simulink library "ammclib_bam_S32K14x"  (R2016a)
settings: Solver=VariableStepAuto  SolverMode=SingleTasking  StartTime=0.0  StopTime=10.0  RelTol=1e-3
undefined symbols (not defined in the file or in its folder): f16A1, f16A2, f16ADCMaxError, f16B0, f16B1, f16B2, f16C1, f16CC1, f16CC1sc, f16CC1sc_D, f16CC1sc_Q, f16CC2, f16CC2sc, f16CC2sc_D, f16CC2sc_Q, f16DerivGain, f16EGain, f16FiltCoef, f16HystOff, f16HystOn, f16IGain, f16IntegGain, f16IntegGainFW, f16IntegGainQ, f16Kd, f16Kq, f16Limit, f16LowerLimit, f16LowerLimit_D, f16LowerLimit_Q, f16LowerLimitFW, f16LowerLimitQ, f16ModIndex, f16OutValOff, f16OutValOn, f16PropGain, f16PropGainFW, f16PropGainQ, f16RampDown, f16RampUp, f16UGain, f16UpperLimit, f16UpperLimit_D, f16UpperLimit_Q, f16UpperLimitFW, f16UpperLimitQ, f16WIGain, f32A1, f32A2, f32ADCMaxError, f32B0, f32B1, f32B2, f32C1, f32CC1, f32CC1sc, f32CC1sc_D, f32CC1sc_Q, f32CC2, f32CC2sc ... (+114)
(part 17 of 22)

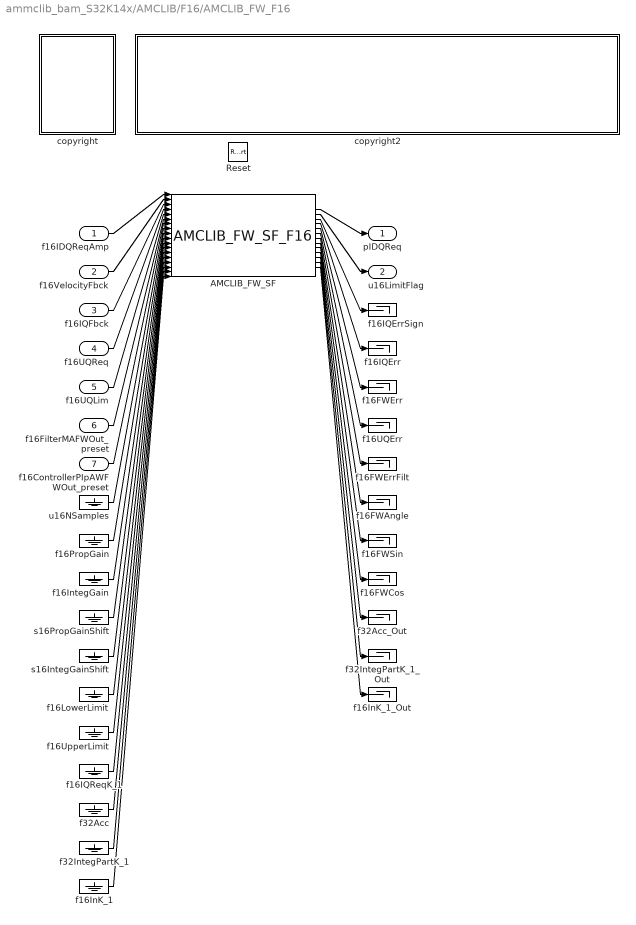
== system ammclib_bam_S32K14x/AMCLIB/F16/AMCLIB_FW_F16 ==
  f16IDQReqAmp : Inport  OutDataTypeStr=int16
  f16VelocityFbck : Inport  Port=2  OutDataTypeStr=int16
  f16IQFbck : Inport  Port=3  OutDataTypeStr=int16
  f16UQReq : Inport  Port=4  OutDataTypeStr=int16
  f16UQLim : Inport  Port=5  OutDataTypeStr=int16
  f16FilterMAFWOut_preset : Inport  Port=6  OutDataTypeStr=int16
  f16ControllerPIpAWFWOut_preset : Inport  Port=7  OutDataTypeStr=int16
  Reset : ResetPort  DisableCoverage=on
  AMCLIB_FW_SF : S-Function  FunctionName=AMCLIB_FW_SF_F16  Parameters=showStates,resetStatesEnable,showDebugOutputs,u16NSamples,f16PropGain,f16IntegGain,s16PropGainShift,s16IntegGainShift,f16LowerLimit,f16UpperLimit  SFunctionDeploymentMode=off  EnableBusSupport=off
  copyright : Subsystem
      mask Display: text(10,90,'FILE:');text(10,75,'DESRIPTION:');text(10,60,'COPYRIGHT:');text(10,45,'VERSION:');text(10,30,'DATE:')
  copyright2 : Subsystem
      mask Display: text(10,90,'AMCLIB_FW_BAM_F16.mdl');text(10,75,'PMSM Field Weakening Controller');text(10,60,'NXP 2020');text(10,45,'1.0');text(10,30,'28-Mar-2020');
  f16FWAngle : Terminator
  f16FWCos : Terminator
  f16FWErr : Terminator
  f16FWErrFilt : Terminator
  f16FWSin : Terminator
  f16IQErr : Terminator
  f16IQErrSign : Terminator
  f16IQReqK_1 : Ground
  f16InK_1 : Ground
  f16InK_1_Out : Terminator
  f16IntegGain : Ground
  f16LowerLimit : Ground
  f16PropGain : Ground
  f16UQErr : Terminator
  f16UpperLimit : Ground
  f32Acc : Ground
  f32Acc_Out : Terminator
  f32IntegPartK_1 : Ground
  f32IntegPartK_1_Out : Terminator
  s16IntegGainShift : Ground
  s16PropGainShift : Ground
  u16NSamples : Ground
  pIDQReq : Outport
  u16LimitFlag : Outport  Port=2
  wires:
  AMCLIB_FW_SF/13 -> f16InK_1_Out/1
  AMCLIB_FW_SF/12 -> f32IntegPartK_1_Out/1
  AMCLIB_FW_SF/11 -> f32Acc_Out/1
  AMCLIB_FW_SF/10 -> f16FWCos/1
  AMCLIB_FW_SF/9 -> f16FWSin/1
  AMCLIB_FW_SF/8 -> f16FWAngle/1
  AMCLIB_FW_SF/7 -> f16FWErrFilt/1
  AMCLIB_FW_SF/6 -> f16UQErr/1
  AMCLIB_FW_SF/5 -> f16FWErr/1
  AMCLIB_FW_SF/4 -> f16IQErr/1
  AMCLIB_FW_SF/3 -> f16IQErrSign/1
  AMCLIB_FW_SF/2 -> u16LimitFlag/1
  AMCLIB_FW_SF/1 -> pIDQReq/1
  f16InK_1/1 -> AMCLIB_FW_SF/18
  f32IntegPartK_1/1 -> AMCLIB_FW_SF/17
  f32Acc/1 -> AMCLIB_FW_SF/16
  f16IQReqK_1/1 -> AMCLIB_FW_SF/15
  f16UpperLimit/1 -> AMCLIB_FW_SF/14
  f16LowerLimit/1 -> AMCLIB_FW_SF/13
  s16IntegGainShift/1 -> AMCLIB_FW_SF/12
  s16PropGainShift/1 -> AMCLIB_FW_SF/11
  f16IntegGain/1 -> AMCLIB_FW_SF/10
  f16PropGain/1 -> AMCLIB_FW_SF/9
  u16NSamples/1 -> AMCLIB_FW_SF/8
  f16ControllerPIpAWFWOut_preset/1 -> AMCLIB_FW_SF/7
  f16FilterMAFWOut_preset/1 -> AMCLIB_FW_SF/6
  f16UQLim/1 -> AMCLIB_FW_SF/5
  f16UQReq/1 -> AMCLIB_FW_SF/4
  f16IQFbck/1 -> AMCLIB_FW_SF/3
  f16VelocityFbck/1 -> AMCLIB_FW_SF/2
  f16IDQReqAmp/1 -> AMCLIB_FW_SF/1

== system ammclib_bam_S32K14x/AMCLIB/F16/AMCLIB_SpeedLoop_F16 ==
  f16VelocityReq : Inport  OutDataTypeStr=int16
  f16VelocityFbck : Inport  Port=2  OutDataTypeStr=int16
  f16FilterMAWOut_preset : Inport  Port=3  OutDataTypeStr=int16
  f16ControllerPIpAWQOut_preset : Inport  Port=4  OutDataTypeStr=int16
  f32RampOut_preset : Inport  Port=5  OutDataTypeStr=int32
  Reset : ResetPort  DisableCoverage=on
  AMCLIB_SpeedLoop_SF : S-Function  FunctionName=AMCLIB_SpeedLoop_SF_F16  Parameters=showStates,resetStatesEnable,showDebugOutputs,u16NSamplesW,f16PropGainQ,f16IntegGainQ,s16PropGainShiftQ,s16IntegGainShiftQ,f16LowerLimitQ,f16UpperLimitQ,f32RampUp,f32RampDown  SFunctionDeploymentMode=off  EnableBusSupport=off
  copyright : Subsystem
      mask Display: text(10,90,'FILE:');text(10,75,'DESRIPTION:');text(10,60,'COPYRIGHT:');text(10,45,'VERSION:');text(10,30,'DATE:')
  copyright2 : Subsystem
      mask Display: text(10,90,'AMCLIB_SpeedLoop_BAM_F16.mdl');text(10,75,'PMSM Speed Loop Controller.');text(10,60,'NXP 2020');text(10,45,'1.0');text(10,30,'28-Mar-2020');
  f16InK_1Q : Ground
  f16InK_1Q_Out : Terminator
  f16IntegGainQ : Ground
  f16LowerLimitQ : Ground
  f16PropGainQ : Ground
  f16UpperLimitQ : Ground
  f16WErr : Terminator
  f16WFbckFilt : Terminator
  f16WReqFilt : Terminator
  f32AccW : Ground
  f32AccW_Out : Terminator
  f32IntegPartK_1Q : Ground
  f32IntegPartK_1Q_Out : Terminator
  f32RampDown : Ground
  f32RampUp : Ground
  f32State : Ground
  f32State_Out : Terminator
  s16IntegGainShiftQ : Ground
  s16PropGainShiftQ : Ground
  u16NSamplesW : Ground
  pIDQReq : Outport
  u16LimitFlagQ : Outport  Port=2
  wires:
  AMCLIB_SpeedLoop_SF/9 -> f32State_Out/1
  AMCLIB_SpeedLoop_SF/8 -> f16InK_1Q_Out/1
  AMCLIB_SpeedLoop_SF/7 -> f32IntegPartK_1Q_Out/1
  AMCLIB_SpeedLoop_SF/6 -> f32AccW_Out/1
  AMCLIB_SpeedLoop_SF/5 -> f16WFbckFilt/1
  AMCLIB_SpeedLoop_SF/4 -> f16WErr/1
  AMCLIB_SpeedLoop_SF/3 -> f16WReqFilt/1
  AMCLIB_SpeedLoop_SF/2 -> u16LimitFlagQ/1
  AMCLIB_SpeedLoop_SF/1 -> pIDQReq/1
  f32State/1 -> AMCLIB_SpeedLoop_SF/18
  f16InK_1Q/1 -> AMCLIB_SpeedLoop_SF/17
  f32IntegPartK_1Q/1 -> AMCLIB_SpeedLoop_SF/16
  f32AccW/1 -> AMCLIB_SpeedLoop_SF/15
  f32RampDown/1 -> AMCLIB_SpeedLoop_SF/14
  f32RampUp/1 -> AMCLIB_SpeedLoop_SF/13
  f16UpperLimitQ/1 -> AMCLIB_SpeedLoop_SF/12
  f16LowerLimitQ/1 -> AMCLIB_SpeedLoop_SF/11
  s16IntegGainShiftQ/1 -> AMCLIB_SpeedLoop_SF/10
  s16PropGainShiftQ/1 -> AMCLIB_SpeedLoop_SF/9
  f16IntegGainQ/1 -> AMCLIB_SpeedLoop_SF/8
  f16PropGainQ/1 -> AMCLIB_SpeedLoop_SF/7
  u16NSamplesW/1 -> AMCLIB_SpeedLoop_SF/6
  f32RampOut_preset/1 -> AMCLIB_SpeedLoop_SF/5
  f16ControllerPIpAWQOut_preset/1 -> AMCLIB_SpeedLoop_SF/4
  f16FilterMAWOut_preset/1 -> AMCLIB_SpeedLoop_SF/3
  f16VelocityFbck/1 -> AMCLIB_SpeedLoop_SF/2
  f16VelocityReq/1 -> AMCLIB_SpeedLoop_SF/1

== system ammclib_bam_S32K14x/AMCLIB/F16/AMCLIB_TrackObsrv_F16 ==
  f16PhaseErr : Inport  OutDataTypeStr=int16
  f16VelocityOut_preset : Inport  Port=2  OutDataTypeStr=int16
  f16PosOut_preset : Inport  Port=3  OutDataTypeStr=int16
  Reset : ResetPort  DisableCoverage=on
  AMCLIB_TrackObsrv_SF : S-Function  FunctionName=AMCLIB_TrackObsrv_SF_F16  Parameters=showStates,resetStatesEnable,f16CC1sc,f16CC2sc,f16UpperLimit,f16LowerLimit,u16NShiftPI,f16C1,u16NShiftI  SFunctionDeploymentMode=off  EnableBusSupport=off
  copyright : Subsystem
      mask Display: text(10,90,'FILE:');text(10,75,'DESRIPTION:');text(10,60,'COPYRIGHT:');text(10,45,'VERSION:');text(10,30,'DATE:')
  copyright2 : Subsystem
      mask Display: text(10,90,'AMCLIB_TrackObsrv_BAM_F16.mdl');text(10,75,'Tracking observer');text(10,60,'NXP 2020');text(10,45,'1.0');text(10,30,'28-Mar-2020');
  f16C1 : Ground
  f16CC1sc : Ground
  f16CC2sc : Ground
  f16InErrK1 : Ground
  f16InErrK1_Out : Terminator
  f16InK1 : Ground
  f16InK1_Out : Terminator
  f16LowerLimit : Ground
  f16UpperLimit : Ground
  f32Acc : Ground
  f32Acc_Out : Terminator
  f32State : Ground
  f32State_Out : Terminator
  u16NShiftI : Ground
  u16NShiftPI : Ground
  pPosEst : Outport
  pVelocityEst : Outport  Port=2
  wires:
  AMCLIB_TrackObsrv_SF/6 -> f16InK1_Out/1
  AMCLIB_TrackObsrv_SF/5 -> f32State_Out/1
  AMCLIB_TrackObsrv_SF/4 -> f16InErrK1_Out/1
  AMCLIB_TrackObsrv_SF/3 -> f32Acc_Out/1
  AMCLIB_TrackObsrv_SF/2 -> pVelocityEst/1
  AMCLIB_TrackObsrv_SF/1 -> pPosEst/1
  f16InK1/1 -> AMCLIB_TrackObsrv_SF/14
  f32State/1 -> AMCLIB_TrackObsrv_SF/13
  f16InErrK1/1 -> AMCLIB_TrackObsrv_SF/12
  f32Acc/1 -> AMCLIB_TrackObsrv_SF/11
  u16NShiftI/1 -> AMCLIB_TrackObsrv_SF/10
  f16C1/1 -> AMCLIB_TrackObsrv_SF/9
  u16NShiftPI/1 -> AMCLIB_TrackObsrv_SF/8
  f16LowerLimit/1 -> AMCLIB_TrackObsrv_SF/7
  f16UpperLimit/1 -> AMCLIB_TrackObsrv_SF/6
  f16CC2sc/1 -> AMCLIB_TrackObsrv_SF/5
  f16CC1sc/1 -> AMCLIB_TrackObsrv_SF/4
  f16PosOut_preset/1 -> AMCLIB_TrackObsrv_SF/3
  f16VelocityOut_preset/1 -> AMCLIB_TrackObsrv_SF/2
  f16PhaseErr/1 -> AMCLIB_TrackObsrv_SF/1

== system ammclib_bam_S32K14x/AMCLIB/F16/AMCLIB_Windmilling_F16 ==
  pUabcIn : Inport  OutDataTypeStr=Bus: SWLIBS_3Syst_F16  BusOutputAsStruct=on
  AMCLIB_Windmilling_SF : S-Function  FunctionName=AMCLIB_Windmilling_SF_F16  Parameters=showStates,f16ADCMaxError,f16CC1sc,f16CC2sc,f16UpperLimit,f16LowerLimit,u16NShiftPI,f16C1,u16NShiftI  SFunctionDeploymentMode=off  EnableBusSupport=off
  copyright : Subsystem
      mask Display: text(10,90,'FILE:');text(10,75,'DESRIPTION:');text(10,60,'COPYRIGHT:');text(10,45,'VERSION:');text(10,30,'DATE:')
  copyright2 : Subsystem
      mask Display: text(10,90,'AMCLIB_Windmilling_BAM_F16.mdl');text(10,75,'PMSM Windmilling');text(10,60,'NXP 2020');text(10,45,'1.0');text(10,30,'28-Mar-2020');
  f16ADCMaxError : Ground
  f16C1 : Ground
  f16CC1sc : Ground
  f16CC2sc : Ground
  f16InErrK1 : Ground
  f16InErrK1_Out : Terminator
  f16InK1 : Ground
  f16InK1_Out : Terminator
  f16LowerLimit : Ground
  f16UpperLimit : Ground
  f32AccPI : Ground
  f32AccPI_Out : Terminator
  f32State : Ground
  f32State_Out : Terminator
  u16NShiftI : Ground
  u16NShiftPI : Ground
  u16Lock : Outport
  pPosEst : Outport  Port=2
  pVelocityEst : Outport  Port=3
  wires:
  AMCLIB_Windmilling_SF/7 -> f16InK1_Out/1
  AMCLIB_Windmilling_SF/6 -> f32State_Out/1
  AMCLIB_Windmilling_SF/5 -> f16InErrK1_Out/1
  AMCLIB_Windmilling_SF/4 -> f32AccPI_Out/1
  AMCLIB_Windmilling_SF/3 -> pVelocityEst/1
  AMCLIB_Windmilling_SF/2 -> pPosEst/1
  AMCLIB_Windmilling_SF/1 -> u16Lock/1
  f16InK1/1 -> AMCLIB_Windmilling_SF/13
  f32State/1 -> AMCLIB_Windmilling_SF/12
  f16InErrK1/1 -> AMCLIB_Windmilling_SF/11
  f32AccPI/1 -> AMCLIB_Windmilling_SF/10
  u16NShiftI/1 -> AMCLIB_Windmilling_SF/9
  f16C1/1 -> AMCLIB_Windmilling_SF/8
  u16NShiftPI/1 -> AMCLIB_Windmilling_SF/7
  f16LowerLimit/1 -> AMCLIB_Windmilling_SF/6
  f16UpperLimit/1 -> AMCLIB_Windmilling_SF/5
  f16CC2sc/1 -> AMCLIB_Windmilling_SF/4
  f16CC1sc/1 -> AMCLIB_Windmilling_SF/3
  f16ADCMaxError/1 -> AMCLIB_Windmilling_SF/2
  pUabcIn/1 -> AMCLIB_Windmilling_SF/1

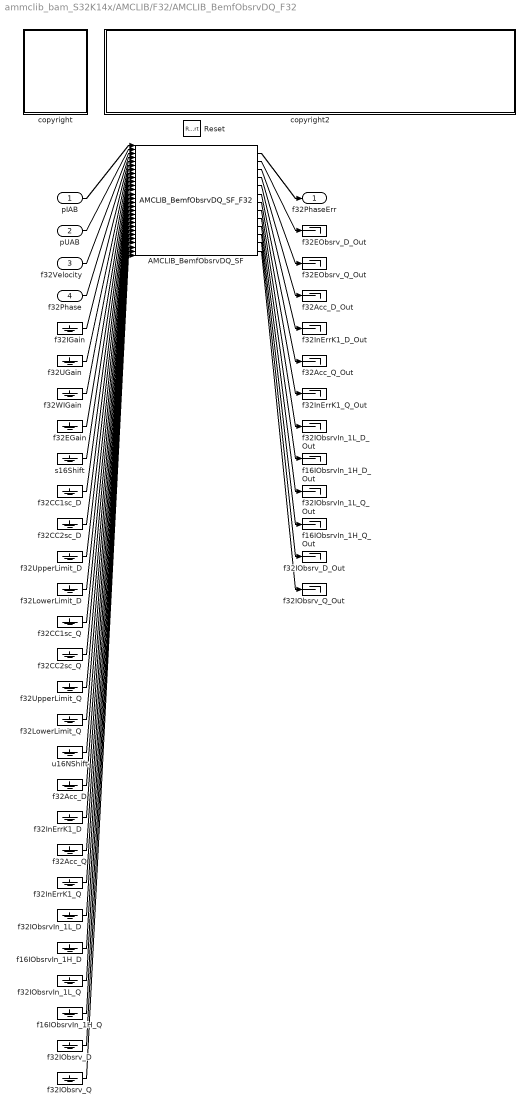
== system ammclib_bam_S32K14x/AMCLIB/F32/AMCLIB_BemfObsrvDQ_F32 ==
  pIAB : Inport  OutDataTypeStr=Bus: SWLIBS_2Syst_F32  BusOutputAsStruct=on
  pUAB : Inport  Port=2  OutDataTypeStr=Bus: SWLIBS_2Syst_F32  BusOutputAsStruct=on
  f32Velocity : Inport  Port=3  OutDataTypeStr=int32
  f32Phase : Inport  Port=4  OutDataTypeStr=int32
  Reset : ResetPort  DisableCoverage=on
  AMCLIB_BemfObsrvDQ_SF : S-Function  FunctionName=AMCLIB_BemfObsrvDQ_SF_F32  Parameters=showStates,resetStatesEnable,f32IGain,f32UGain,f32WIGain,f32EGain,s16Shift,f32CC1sc_D,f32CC2sc_D,f32UpperLimit_D,f32LowerLimit_D,f32CC1sc_Q,f32CC2sc_Q,f32UpperLimit_Q,f32LowerLimit_Q,u16NShift  SFunctionDeploymentMode=off  EnableBusSupport=off
  copyright : Subsystem
      mask Display: text(10,90,'FILE:');text(10,75,'DESRIPTION:');text(10,60,'COPYRIGHT:');text(10,45,'VERSION:');text(10,30,'DATE:')
  copyright2 : Subsystem
      mask Display: text(10,90,'AMCLIB_BemfObsrvDQ_BAM_F32.mdl');text(10,75,'PMSM back-EMF observer DQ.');text(10,60,'NXP 2020');text(10,45,'1.0');text(10,30,'28-Mar-2020');
  f16IObsrvIn_1H_D : Ground
  f16IObsrvIn_1H_D_Out : Terminator
  f16IObsrvIn_1H_Q : Ground
  f16IObsrvIn_1H_Q_Out : Terminator
  f32Acc_D : Ground
  f32Acc_D_Out : Terminator
  f32Acc_Q : Ground
  f32Acc_Q_Out : Terminator
  f32CC1sc_D : Ground
  f32CC1sc_Q : Ground
  f32CC2sc_D : Ground
  f32CC2sc_Q : Ground
  f32EGain : Ground
  f32EObsrv_D_Out : Terminator
  f32EObsrv_Q_Out : Terminator
  f32IGain : Ground
  f32IObsrvIn_1L_D : Ground
  f32IObsrvIn_1L_D_Out : Terminator
  f32IObsrvIn_1L_Q : Ground
  f32IObsrvIn_1L_Q_Out : Terminator
  f32IObsrv_D : Ground
  f32IObsrv_D_Out : Terminator
  f32IObsrv_Q : Ground
  f32IObsrv_Q_Out : Terminator
  f32InErrK1_D : Ground
  f32InErrK1_D_Out : Terminator
  f32InErrK1_Q : Ground
  f32InErrK1_Q_Out : Terminator
  f32LowerLimit_D : Ground
  f32LowerLimit_Q : Ground
  f32UGain : Ground
  f32UpperLimit_D : Ground
  f32UpperLimit_Q : Ground
  f32WIGain : Ground
  s16Shift : Ground
  u16NShift : Ground
  f32PhaseErr : Outport
  wires:
  AMCLIB_BemfObsrvDQ_SF/13 -> f32IObsrv_Q_Out/1
  AMCLIB_BemfObsrvDQ_SF/12 -> f32IObsrv_D_Out/1
  AMCLIB_BemfObsrvDQ_SF/11 -> f16IObsrvIn_1H_Q_Out/1
  AMCLIB_BemfObsrvDQ_SF/10 -> f32IObsrvIn_1L_Q_Out/1
  AMCLIB_BemfObsrvDQ_SF/9 -> f16IObsrvIn_1H_D_Out/1
  AMCLIB_BemfObsrvDQ_SF/8 -> f32IObsrvIn_1L_D_Out/1
  AMCLIB_BemfObsrvDQ_SF/7 -> f32InErrK1_Q_Out/1
  AMCLIB_BemfObsrvDQ_SF/6 -> f32Acc_Q_Out/1
  AMCLIB_BemfObsrvDQ_SF/5 -> f32InErrK1_D_Out/1
  AMCLIB_BemfObsrvDQ_SF/4 -> f32Acc_D_Out/1
  AMCLIB_BemfObsrvDQ_SF/3 -> f32EObsrv_Q_Out/1
  AMCLIB_BemfObsrvDQ_SF/2 -> f32EObsrv_D_Out/1
  AMCLIB_BemfObsrvDQ_SF/1 -> f32PhaseErr/1
  f32IObsrv_Q/1 -> AMCLIB_BemfObsrvDQ_SF/28
  f32IObsrv_D/1 -> AMCLIB_BemfObsrvDQ_SF/27
  f16IObsrvIn_1H_Q/1 -> AMCLIB_BemfObsrvDQ_SF/26
  f32IObsrvIn_1L_Q/1 -> AMCLIB_BemfObsrvDQ_SF/25
  f16IObsrvIn_1H_D/1 -> AMCLIB_BemfObsrvDQ_SF/24
  f32IObsrvIn_1L_D/1 -> AMCLIB_BemfObsrvDQ_SF/23
  f32InErrK1_Q/1 -> AMCLIB_BemfObsrvDQ_SF/22
  f32Acc_Q/1 -> AMCLIB_BemfObsrvDQ_SF/21
  f32InErrK1_D/1 -> AMCLIB_BemfObsrvDQ_SF/20
  f32Acc_D/1 -> AMCLIB_BemfObsrvDQ_SF/19
  u16NShift/1 -> AMCLIB_BemfObsrvDQ_SF/18
  f32LowerLimit_Q/1 -> AMCLIB_BemfObsrvDQ_SF/17
  f32UpperLimit_Q/1 -> AMCLIB_BemfObsrvDQ_SF/16
  f32CC2sc_Q/1 -> AMCLIB_BemfObsrvDQ_SF/15
  f32CC1sc_Q/1 -> AMCLIB_BemfObsrvDQ_SF/14
  f32LowerLimit_D/1 -> AMCLIB_BemfObsrvDQ_SF/13
  f32UpperLimit_D/1 -> AMCLIB_BemfObsrvDQ_SF/12
  f32CC2sc_D/1 -> AMCLIB_BemfObsrvDQ_SF/11
  f32CC1sc_D/1 -> AMCLIB_BemfObsrvDQ_SF/10
  s16Shift/1 -> AMCLIB_BemfObsrvDQ_SF/9
  f32EGain/1 -> AMCLIB_BemfObsrvDQ_SF/8
  f32WIGain/1 -> AMCLIB_BemfObsrvDQ_SF/7
  f32UGain/1 -> AMCLIB_BemfObsrvDQ_SF/6
  f32IGain/1 -> AMCLIB_BemfObsrvDQ_SF/5
  f32Phase/1 -> AMCLIB_BemfObsrvDQ_SF/4
  f32Velocity/1 -> AMCLIB_BemfObsrvDQ_SF/3
  pUAB/1 -> AMCLIB_BemfObsrvDQ_SF/2
  pIAB/1 -> AMCLIB_BemfObsrvDQ_SF/1

== system ammclib_bam_S32K14x/AMCLIB/F32/AMCLIB_CurrentLoop_F32 ==
  f32UDcBus : Inport  OutDataTypeStr=int32
  pIDQReq : Inport  Port=2  OutDataTypeStr=Bus: SWLIBS_2Syst_F32  BusOutputAsStruct=on
  pIDQFbck : Inport  Port=3  OutDataTypeStr=Bus: SWLIBS_2Syst_F32  BusOutputAsStruct=on
  f32ControllerPIrAWDOut_preset : Inport  Port=4  OutDataTypeStr=int32
  f32ControllerPIrAWQOut_preset : Inport  Port=5  OutDataTypeStr=int32
  Reset : ResetPort  DisableCoverage=on
  AMCLIB_CurrentLoop_SF : S-Function  FunctionName=AMCLIB_CurrentLoop_SF_F32  Parameters=showStates,resetStatesEnable,f32CC1sc_D,f32CC2sc_D,u16NShift_D,f32CC1sc_Q,f32CC2sc_Q,u16NShift_Q  SFunctionDeploymentMode=off  EnableBusSupport=off
  copyright : Subsystem
      mask Display: text(10,90,'FILE:');text(10,75,'DESRIPTION:');text(10,60,'COPYRIGHT:');text(10,45,'VERSION:');text(10,30,'DATE:')
  copyright2 : Subsystem
      mask Display: text(10,90,'AMCLIB_CurrentLoop_BAM_F32.mdl');text(10,75,'PMSM Current Loop.');text(10,60,'NXP 2020');text(10,45,'1.0');text(10,30,'28-Mar-2020');
  f32Acc_D : Ground
  f32Acc_D_Out : Terminator
  f32Acc_Q : Ground
  f32Acc_Q_Out : Terminator
  f32CC1sc_D : Ground
  f32CC1sc_Q : Ground
  f32CC2sc_D : Ground
  f32CC2sc_Q : Ground
  f32InErrK1_D : Ground
  f32InErrK1_D_Out : Terminator
  f32InErrK1_Q : Ground
  f32InErrK1_Q_Out : Terminator
  u16NShift_D : Ground
  u16NShift_Q : Ground
  pUDQReq : Outport
  wires:
  AMCLIB_CurrentLoop_SF/5 -> f32InErrK1_Q_Out/1
  AMCLIB_CurrentLoop_SF/4 -> f32Acc_Q_Out/1
  AMCLIB_CurrentLoop_SF/3 -> f32InErrK1_D_Out/1
  AMCLIB_CurrentLoop_SF/2 -> f32Acc_D_Out/1
  AMCLIB_CurrentLoop_SF/1 -> pUDQReq/1
  f32InErrK1_Q/1 -> AMCLIB_CurrentLoop_SF/15
  f32Acc_Q/1 -> AMCLIB_CurrentLoop_SF/14
  f32InErrK1_D/1 -> AMCLIB_CurrentLoop_SF/13
  f32Acc_D/1 -> AMCLIB_CurrentLoop_SF/12
  u16NShift_Q/1 -> AMCLIB_CurrentLoop_SF/11
  f32CC2sc_Q/1 -> AMCLIB_CurrentLoop_SF/10
  f32CC1sc_Q/1 -> AMCLIB_CurrentLoop_SF/9
  u16NShift_D/1 -> AMCLIB_CurrentLoop_SF/8
  f32CC2sc_D/1 -> AMCLIB_CurrentLoop_SF/7
  f32CC1sc_D/1 -> AMCLIB_CurrentLoop_SF/6
  f32ControllerPIrAWQOut_preset/1 -> AMCLIB_CurrentLoop_SF/5
  f32ControllerPIrAWDOut_preset/1 -> AMCLIB_CurrentLoop_SF/4
  pIDQFbck/1 -> AMCLIB_CurrentLoop_SF/3
  pIDQReq/1 -> AMCLIB_CurrentLoop_SF/2
  f32UDcBus/1 -> AMCLIB_CurrentLoop_SF/1

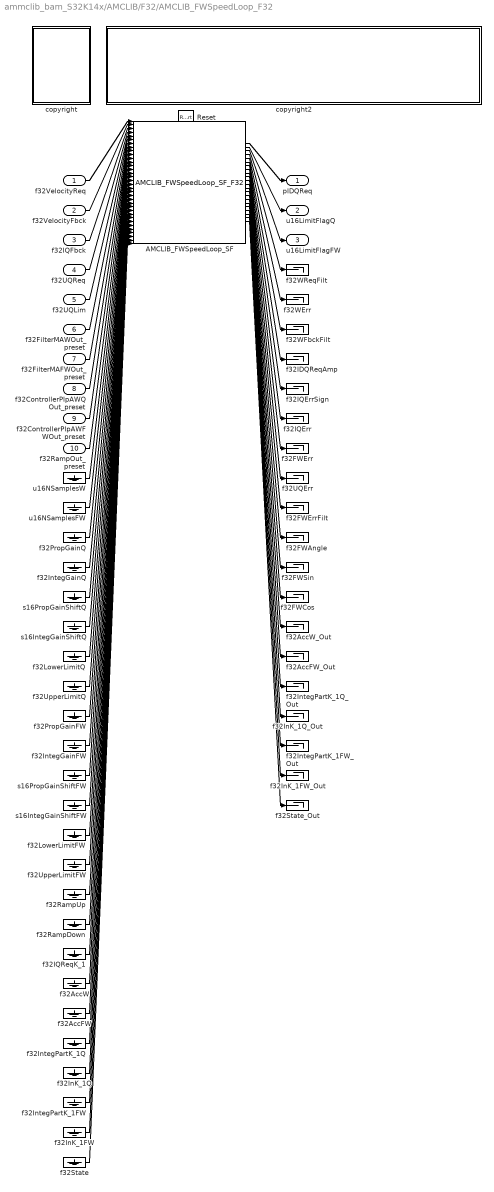
== system ammclib_bam_S32K14x/AMCLIB/F32/AMCLIB_FWSpeedLoop_F32 ==
  f32VelocityReq : Inport  OutDataTypeStr=int32
  f32VelocityFbck : Inport  Port=2  OutDataTypeStr=int32
  f32IQFbck : Inport  Port=3  OutDataTypeStr=int32
  f32UQReq : Inport  Port=4  OutDataTypeStr=int32
  f32UQLim : Inport  Port=5  OutDataTypeStr=int32
  f32FilterMAWOut_preset : Inport  Port=6  OutDataTypeStr=int32
  f32FilterMAFWOut_preset : Inport  Port=7  OutDataTypeStr=int32
  f32ControllerPIpAWQOut_preset : Inport  Port=8  OutDataTypeStr=int32
  f32ControllerPIpAWFWOut_preset : Inport  Port=9  OutDataTypeStr=int32
  f32RampOut_preset : Inport  Port=10  OutDataTypeStr=int32
  Reset : ResetPort  DisableCoverage=on
  AMCLIB_FWSpeedLoop_SF : S-Function  FunctionName=AMCLIB_FWSpeedLoop_SF_F32  Parameters=showStates,resetStatesEnable,showDebugOutputs,u16NSamplesW,u16NSamplesFW,f32PropGainQ,f32IntegGainQ,s16PropGainShiftQ,s16IntegGainShiftQ,f32LowerLimitQ,f32UpperLimitQ,f32PropGainFW,f32IntegGainFW,s16PropGainShiftFW,s16IntegGainShiftFW,f32LowerLimitFW,f32UpperLimitFW,f32RampUp,f32RampDown  SFunctionDeploymentMode=off  EnableBusSupport=off
  copyright : Subsystem
      mask Display: text(10,90,'FILE:');text(10,75,'DESRIPTION:');text(10,60,'COPYRIGHT:');text(10,45,'VERSION:');text(10,30,'DATE:')
  copyright2 : Subsystem
      mask Display: text(10,90,'AMCLIB_FWSpeedLoop_BAM_F32.mdl');text(10,75,'PMSM Speed Loop with Field Weakening.');text(10,60,'NXP 2020');text(10,45,'1.0');text(10,30,'28-Mar-2020');
  f32AccFW : Ground
  f32AccFW_Out : Terminator
  f32AccW : Ground
  f32AccW_Out : Terminator
  f32FWAngle : Terminator
  f32FWCos : Terminator
  f32FWErr : Terminator
  f32FWErrFilt : Terminator
  f32FWSin : Terminator
  f32IDQReqAmp : Terminator
  f32IQErr : Terminator
  f32IQErrSign : Terminator
  f32IQReqK_1 : Ground
  f32InK_1FW : Ground
  f32InK_1FW_Out : Terminator
  f32InK_1Q : Ground
  f32InK_1Q_Out : Terminator
  f32IntegGainFW : Ground
  f32IntegGainQ : Ground
  f32IntegPartK_1FW : Ground
  f32IntegPartK_1FW_Out : Terminator
  f32IntegPartK_1Q : Ground
  f32IntegPartK_1Q_Out : Terminator
  f32LowerLimitFW : Ground
  f32LowerLimitQ : Ground
  f32PropGainFW : Ground
  f32PropGainQ : Ground
  f32RampDown : Ground
  f32RampUp : Ground
  f32State : Ground
  f32State_Out : Terminator
  f32UQErr : Terminator
  f32UpperLimitFW : Ground
  f32UpperLimitQ : Ground
  f32WErr : Terminator
  f32WFbckFilt : Terminator
  f32WReqFilt : Terminator
  s16IntegGainShiftFW : Ground
  s16IntegGainShiftQ : Ground
  s16PropGainShiftFW : Ground
  s16PropGainShiftQ : Ground
  u16NSamplesFW : Ground
  u16NSamplesW : Ground
  pIDQReq : Outport
  u16LimitFlagQ : Outport  Port=2
  u16LimitFlagFW : Outport  Port=3
  wires:
  AMCLIB_FWSpeedLoop_SF/22 -> f32State_Out/1
  AMCLIB_FWSpeedLoop_SF/21 -> f32InK_1FW_Out/1
  AMCLIB_FWSpeedLoop_SF/20 -> f32IntegPartK_1FW_Out/1
  AMCLIB_FWSpeedLoop_SF/19 -> f32InK_1Q_Out/1
  AMCLIB_FWSpeedLoop_SF/18 -> f32IntegPartK_1Q_Out/1
  AMCLIB_FWSpeedLoop_SF/17 -> f32AccFW_Out/1
  AMCLIB_FWSpeedLoop_SF/16 -> f32AccW_Out/1
  AMCLIB_FWSpeedLoop_SF/15 -> f32FWCos/1
  AMCLIB_FWSpeedLoop_SF/14 -> f32FWSin/1
  AMCLIB_FWSpeedLoop_SF/13 -> f32FWAngle/1
  AMCLIB_FWSpeedLoop_SF/12 -> f32FWErrFilt/1
  AMCLIB_FWSpeedLoop_SF/11 -> f32UQErr/1
  AMCLIB_FWSpeedLoop_SF/10 -> f32FWErr/1
  AMCLIB_FWSpeedLoop_SF/9 -> f32IQErr/1
  AMCLIB_FWSpeedLoop_SF/8 -> f32IQErrSign/1
  AMCLIB_FWSpeedLoop_SF/7 -> f32IDQReqAmp/1
  AMCLIB_FWSpeedLoop_SF/6 -> f32WFbckFilt/1
  AMCLIB_FWSpeedLoop_SF/5 -> f32WErr/1
  AMCLIB_FWSpeedLoop_SF/4 -> f32WReqFilt/1
  AMCLIB_FWSpeedLoop_SF/3 -> u16LimitFlagFW/1
  AMCLIB_FWSpeedLoop_SF/2 -> u16LimitFlagQ/1
  AMCLIB_FWSpeedLoop_SF/1 -> pIDQReq/1
  f32State/1 -> AMCLIB_FWSpeedLoop_SF/34
  f32InK_1FW/1 -> AMCLIB_FWSpeedLoop_SF/33
  f32IntegPartK_1FW/1 -> AMCLIB_FWSpeedLoop_SF/32
  f32InK_1Q/1 -> AMCLIB_FWSpeedLoop_SF/31
  f32IntegPartK_1Q/1 -> AMCLIB_FWSpeedLoop_SF/30
  f32AccFW/1 -> AMCLIB_FWSpeedLoop_SF/29
  f32AccW/1 -> AMCLIB_FWSpeedLoop_SF/28
  f32IQReqK_1/1 -> AMCLIB_FWSpeedLoop_SF/27
  f32RampDown/1 -> AMCLIB_FWSpeedLoop_SF/26
  f32RampUp/1 -> AMCLIB_FWSpeedLoop_SF/25
  f32UpperLimitFW/1 -> AMCLIB_FWSpeedLoop_SF/24
  f32LowerLimitFW/1 -> AMCLIB_FWSpeedLoop_SF/23
  s16IntegGainShiftFW/1 -> AMCLIB_FWSpeedLoop_SF/22
  s16PropGainShiftFW/1 -> AMCLIB_FWSpeedLoop_SF/21
  f32IntegGainFW/1 -> AMCLIB_FWSpeedLoop_SF/20
  f32PropGainFW/1 -> AMCLIB_FWSpeedLoop_SF/19
  f32UpperLimitQ/1 -> AMCLIB_FWSpeedLoop_SF/18
  f32LowerLimitQ/1 -> AMCLIB_FWSpeedLoop_SF/17
  s16IntegGainShiftQ/1 -> AMCLIB_FWSpeedLoop_SF/16
  s16PropGainShiftQ/1 -> AMCLIB_FWSpeedLoop_SF/15
  f32IntegGainQ/1 -> AMCLIB_FWSpeedLoop_SF/14
  f32PropGainQ/1 -> AMCLIB_FWSpeedLoop_SF/13
  u16NSamplesFW/1 -> AMCLIB_FWSpeedLoop_SF/12
  u16NSamplesW/1 -> AMCLIB_FWSpeedLoop_SF/11
  f32RampOut_preset/1 -> AMCLIB_FWSpeedLoop_SF/10
  f32ControllerPIpAWFWOut_preset/1 -> AMCLIB_FWSpeedLoop_SF/9
  f32ControllerPIpAWQOut_preset/1 -> AMCLIB_FWSpeedLoop_SF/8
  f32FilterMAFWOut_preset/1 -> AMCLIB_FWSpeedLoop_SF/7
  f32FilterMAWOut_preset/1 -> AMCLIB_FWSpeedLoop_SF/6
  f32UQLim/1 -> AMCLIB_FWSpeedLoop_SF/5
  f32UQReq/1 -> AMCLIB_FWSpeedLoop_SF/4
  f32IQFbck/1 -> AMCLIB_FWSpeedLoop_SF/3
  f32VelocityFbck/1 -> AMCLIB_FWSpeedLoop_SF/2
  f32VelocityReq/1 -> AMCLIB_FWSpeedLoop_SF/1

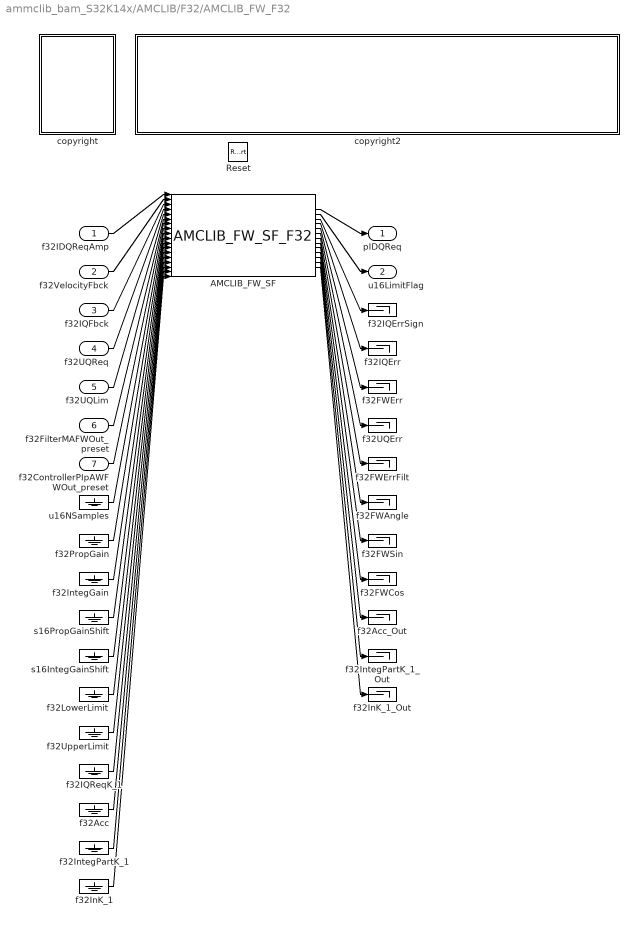
== system ammclib_bam_S32K14x/AMCLIB/F32/AMCLIB_FW_F32 ==
  f32IDQReqAmp : Inport  OutDataTypeStr=int32
  f32VelocityFbck : Inport  Port=2  OutDataTypeStr=int32
  f32IQFbck : Inport  Port=3  OutDataTypeStr=int32
  f32UQReq : Inport  Port=4  OutDataTypeStr=int32
  f32UQLim : Inport  Port=5  OutDataTypeStr=int32
  f32FilterMAFWOut_preset : Inport  Port=6  OutDataTypeStr=int32
  f32ControllerPIpAWFWOut_preset : Inport  Port=7  OutDataTypeStr=int32
  Reset : ResetPort  DisableCoverage=on
  AMCLIB_FW_SF : S-Function  FunctionName=AMCLIB_FW_SF_F32  Parameters=showStates,resetStatesEnable,showDebugOutputs,u16NSamples,f32PropGain,f32IntegGain,s16PropGainShift,s16IntegGainShift,f32LowerLimit,f32UpperLimit  SFunctionDeploymentMode=off  EnableBusSupport=off
  copyright : Subsystem
      mask Display: text(10,90,'FILE:');text(10,75,'DESRIPTION:');text(10,60,'COPYRIGHT:');text(10,45,'VERSION:');text(10,30,'DATE:')
  copyright2 : Subsystem
      mask Display: text(10,90,'AMCLIB_FW_BAM_F32.mdl');text(10,75,'PMSM Field Weakening Controller');text(10,60,'NXP 2020');text(10,45,'1.0');text(10,30,'28-Mar-2020');
  f32Acc : Ground
  f32Acc_Out : Terminator
  f32FWAngle : Terminator
  f32FWCos : Terminator
  f32FWErr : Terminator
  f32FWErrFilt : Terminator
  f32FWSin : Terminator
  f32IQErr : Terminator
  f32IQErrSign : Terminator
  f32IQReqK_1 : Ground
  f32InK_1 : Ground
  f32InK_1_Out : Terminator
  f32IntegGain : Ground
  f32IntegPartK_1 : Ground
  f32IntegPartK_1_Out : Terminator
  f32LowerLimit : Ground
  f32PropGain : Ground
  f32UQErr : Terminator
  f32UpperLimit : Ground
  s16IntegGainShift : Ground
  s16PropGainShift : Ground
  u16NSamples : Ground
  pIDQReq : Outport
  u16LimitFlag : Outport  Port=2
  wires:
  AMCLIB_FW_SF/13 -> f32InK_1_Out/1
  AMCLIB_FW_SF/12 -> f32IntegPartK_1_Out/1
  AMCLIB_FW_SF/11 -> f32Acc_Out/1
  AMCLIB_FW_SF/10 -> f32FWCos/1
  AMCLIB_FW_SF/9 -> f32FWSin/1
  AMCLIB_FW_SF/8 -> f32FWAngle/1
  AMCLIB_FW_SF/7 -> f32FWErrFilt/1
  AMCLIB_FW_SF/6 -> f32UQErr/1
  AMCLIB_FW_SF/5 -> f32FWErr/1
  AMCLIB_FW_SF/4 -> f32IQErr/1
  AMCLIB_FW_SF/3 -> f32IQErrSign/1
  AMCLIB_FW_SF/2 -> u16LimitFlag/1
  AMCLIB_FW_SF/1 -> pIDQReq/1
  f32InK_1/1 -> AMCLIB_FW_SF/18
  f32IntegPartK_1/1 -> AMCLIB_FW_SF/17
  f32Acc/1 -> AMCLIB_FW_SF/16
  f32IQReqK_1/1 -> AMCLIB_FW_SF/15
  f32UpperLimit/1 -> AMCLIB_FW_SF/14
  f32LowerLimit/1 -> AMCLIB_FW_SF/13
  s16IntegGainShift/1 -> AMCLIB_FW_SF/12
  s16PropGainShift/1 -> AMCLIB_FW_SF/11
  f32IntegGain/1 -> AMCLIB_FW_SF/10
  f32PropGain/1 -> AMCLIB_FW_SF/9
  u16NSamples/1 -> AMCLIB_FW_SF/8
  f32ControllerPIpAWFWOut_preset/1 -> AMCLIB_FW_SF/7
  f32FilterMAFWOut_preset/1 -> AMCLIB_FW_SF/6
  f32UQLim/1 -> AMCLIB_FW_SF/5
  f32UQReq/1 -> AMCLIB_FW_SF/4
  f32IQFbck/1 -> AMCLIB_FW_SF/3
  f32VelocityFbck/1 -> AMCLIB_FW_SF/2
  f32IDQReqAmp/1 -> AMCLIB_FW_SF/1

== system ammclib_bam_S32K14x/AMCLIB/F32/AMCLIB_SpeedLoop_F32 ==
  f32VelocityReq : Inport  OutDataTypeStr=int32
  f32VelocityFbck : Inport  Port=2  OutDataTypeStr=int32
  f32FilterMAWOut_preset : Inport  Port=3  OutDataTypeStr=int32
  f32ControllerPIpAWQOut_preset : Inport  Port=4  OutDataTypeStr=int32
  f32RampOut_preset : Inport  Port=5  OutDataTypeStr=int32
  Reset : ResetPort  DisableCoverage=on
  AMCLIB_SpeedLoop_SF : S-Function  FunctionName=AMCLIB_SpeedLoop_SF_F32  Parameters=showStates,resetStatesEnable,showDebugOutputs,u16NSamplesW,f32PropGainQ,f32IntegGainQ,s16PropGainShiftQ,s16IntegGainShiftQ,f32LowerLimitQ,f32UpperLimitQ,f32RampUp,f32RampDown  SFunctionDeploymentMode=off  EnableBusSupport=off
  copyright : Subsystem
      mask Display: text(10,90,'FILE:');text(10,75,'DESRIPTION:');text(10,60,'COPYRIGHT:');text(10,45,'VERSION:');text(10,30,'DATE:')
  copyright2 : Subsystem
      mask Display: text(10,90,'AMCLIB_SpeedLoop_BAM_F32.mdl');text(10,75,'PMSM Speed Loop Controller.');text(10,60,'NXP 2020');text(10,45,'1.0');text(10,30,'28-Mar-2020');
  f32AccW : Ground
  f32AccW_Out : Terminator
  f32InK_1Q : Ground
  f32InK_1Q_Out : Terminator
  f32IntegGainQ : Ground
  f32IntegPartK_1Q : Ground
  f32IntegPartK_1Q_Out : Terminator
  f32LowerLimitQ : Ground
  f32PropGainQ : Ground
  f32RampDown : Ground
  f32RampUp : Ground
  f32State : Ground
  f32State_Out : Terminator
  f32UpperLimitQ : Ground
  f32WErr : Terminator
  f32WFbckFilt : Terminator
  f32WReqFilt : Terminator
  s16IntegGainShiftQ : Ground
  s16PropGainShiftQ : Ground
  u16NSamplesW : Ground
  pIDQReq : Outport
  u16LimitFlagQ : Outport  Port=2
  wires:
  AMCLIB_SpeedLoop_SF/9 -> f32State_Out/1
  AMCLIB_SpeedLoop_SF/8 -> f32InK_1Q_Out/1
  AMCLIB_SpeedLoop_SF/7 -> f32IntegPartK_1Q_Out/1
  AMCLIB_SpeedLoop_SF/6 -> f32AccW_Out/1
  AMCLIB_SpeedLoop_SF/5 -> f32WFbckFilt/1
  AMCLIB_SpeedLoop_SF/4 -> f32WErr/1
  AMCLIB_SpeedLoop_SF/3 -> f32WReqFilt/1
  AMCLIB_SpeedLoop_SF/2 -> u16LimitFlagQ/1
  AMCLIB_SpeedLoop_SF/1 -> pIDQReq/1
  f32State/1 -> AMCLIB_SpeedLoop_SF/18
  f32InK_1Q/1 -> AMCLIB_SpeedLoop_SF/17
  f32IntegPartK_1Q/1 -> AMCLIB_SpeedLoop_SF/16
  f32AccW/1 -> AMCLIB_SpeedLoop_SF/15
  f32RampDown/1 -> AMCLIB_SpeedLoop_SF/14
  f32RampUp/1 -> AMCLIB_SpeedLoop_SF/13
  f32UpperLimitQ/1 -> AMCLIB_SpeedLoop_SF/12
  f32LowerLimitQ/1 -> AMCLIB_SpeedLoop_SF/11
  s16IntegGainShiftQ/1 -> AMCLIB_SpeedLoop_SF/10
  s16PropGainShiftQ/1 -> AMCLIB_SpeedLoop_SF/9
  f32IntegGainQ/1 -> AMCLIB_SpeedLoop_SF/8
  f32PropGainQ/1 -> AMCLIB_SpeedLoop_SF/7
  u16NSamplesW/1 -> AMCLIB_SpeedLoop_SF/6
  f32RampOut_preset/1 -> AMCLIB_SpeedLoop_SF/5
  f32ControllerPIpAWQOut_preset/1 -> AMCLIB_SpeedLoop_SF/4
  f32FilterMAWOut_preset/1 -> AMCLIB_SpeedLoop_SF/3
  f32VelocityFbck/1 -> AMCLIB_SpeedLoop_SF/2
  f32VelocityReq/1 -> AMCLIB_SpeedLoop_SF/1

== system ammclib_bam_S32K14x/AMCLIB/F32/AMCLIB_TrackObsrv_F32 ==
  f32PhaseErr : Inport  OutDataTypeStr=int32
  f32VelocityOut_preset : Inport  Port=2  OutDataTypeStr=int32
  f32PosOut_preset : Inport  Port=3  OutDataTypeStr=int32
  Reset : ResetPort  DisableCoverage=on
  AMCLIB_TrackObsrv_SF : S-Function  FunctionName=AMCLIB_TrackObsrv_SF_F32  Parameters=showStates,resetStatesEnable,f32CC1sc,f32CC2sc,f32UpperLimit,f32LowerLimit,u16NShiftPI,f32C1,u16NShiftI  SFunctionDeploymentMode=off  EnableBusSupport=off
  copyright : Subsystem
      mask Display: text(10,90,'FILE:');text(10,75,'DESRIPTION:');text(10,60,'COPYRIGHT:');text(10,45,'VERSION:');text(10,30,'DATE:')
  copyright2 : Subsystem
      mask Display: text(10,90,'AMCLIB_TrackObsrv_BAM_F32.mdl');text(10,75,'Tracking observer');text(10,60,'NXP 2020');text(10,45,'1.0');text(10,30,'28-Mar-2020');
  f32Acc : Ground
  f32Acc_Out : Terminator
  f32C1 : Ground
  f32CC1sc : Ground
  f32CC2sc : Ground
  f32InErrK1 : Ground
  f32InErrK1_Out : Terminator
  f32InK1 : Ground
  f32InK1_Out : Terminator
  f32LowerLimit : Ground
  f32State : Ground
  f32State_Out : Terminator
  f32UpperLimit : Ground
  u16NShiftI : Ground
  u16NShiftPI : Ground
  pPosEst : Outport
  pVelocityEst : Outport  Port=2
  wires:
  AMCLIB_TrackObsrv_SF/6 -> f32InK1_Out/1
  AMCLIB_TrackObsrv_SF/5 -> f32State_Out/1
  AMCLIB_TrackObsrv_SF/4 -> f32InErrK1_Out/1
  AMCLIB_TrackObsrv_SF/3 -> f32Acc_Out/1
  AMCLIB_TrackObsrv_SF/2 -> pVelocityEst/1
  AMCLIB_TrackObsrv_SF/1 -> pPosEst/1
  f32InK1/1 -> AMCLIB_TrackObsrv_SF/14
  f32State/1 -> AMCLIB_TrackObsrv_SF/13
  f32InErrK1/1 -> AMCLIB_TrackObsrv_SF/12
  f32Acc/1 -> AMCLIB_TrackObsrv_SF/11
  u16NShiftI/1 -> AMCLIB_TrackObsrv_SF/10
  f32C1/1 -> AMCLIB_TrackObsrv_SF/9
  u16NShiftPI/1 -> AMCLIB_TrackObsrv_SF/8
  f32LowerLimit/1 -> AMCLIB_TrackObsrv_SF/7
  f32UpperLimit/1 -> AMCLIB_TrackObsrv_SF/6
  f32CC2sc/1 -> AMCLIB_TrackObsrv_SF/5
  f32CC1sc/1 -> AMCLIB_TrackObsrv_SF/4
  f32PosOut_preset/1 -> AMCLIB_TrackObsrv_SF/3
  f32VelocityOut_preset/1 -> AMCLIB_TrackObsrv_SF/2
  f32PhaseErr/1 -> AMCLIB_TrackObsrv_SF/1

== system ammclib_bam_S32K14x/AMCLIB/F32/AMCLIB_Windmilling_F32 ==
  pUabcIn : Inport  OutDataTypeStr=Bus: SWLIBS_3Syst_F32  BusOutputAsStruct=on
  AMCLIB_Windmilling_SF : S-Function  FunctionName=AMCLIB_Windmilling_SF_F32  Parameters=showStates,f32ADCMaxError,f32CC1sc,f32CC2sc,f32UpperLimit,f32LowerLimit,u16NShiftPI,f32C1,u16NShiftI  SFunctionDeploymentMode=off  EnableBusSupport=off
  copyright : Subsystem
      mask Display: text(10,90,'FILE:');text(10,75,'DESRIPTION:');text(10,60,'COPYRIGHT:');text(10,45,'VERSION:');text(10,30,'DATE:')
  copyright2 : Subsystem
      mask Display: text(10,90,'AMCLIB_Windmilling_BAM_F32.mdl');text(10,75,'PMSM Windmilling');text(10,60,'NXP 2020');text(10,45,'1.0');text(10,30,'28-Mar-2020');
  f32ADCMaxError : Ground
  f32AccPI : Ground
  f32AccPI_Out : Terminator
  f32C1 : Ground
  f32CC1sc : Ground
  f32CC2sc : Ground
  f32InErrK1 : Ground
  f32InErrK1_Out : Terminator
  f32InK1 : Ground
  f32InK1_Out : Terminator
  f32LowerLimit : Ground
  f32State : Ground
  f32State_Out : Terminator
  f32UpperLimit : Ground
  u16NShiftI : Ground
  u16NShiftPI : Ground
  u32Lock : Outport
  pPosEst : Outport  Port=2
  pVelocityEst : Outport  Port=3
  wires:
  AMCLIB_Windmilling_SF/7 -> f32InK1_Out/1
  AMCLIB_Windmilling_SF/6 -> f32State_Out/1
  AMCLIB_Windmilling_SF/5 -> f32InErrK1_Out/1
  AMCLIB_Windmilling_SF/4 -> f32AccPI_Out/1
  AMCLIB_Windmilling_SF/3 -> pVelocityEst/1
  AMCLIB_Windmilling_SF/2 -> pPosEst/1
  AMCLIB_Windmilling_SF/1 -> u32Lock/1
  f32InK1/1 -> AMCLIB_Windmilling_SF/13
  f32State/1 -> AMCLIB_Windmilling_SF/12
  f32InErrK1/1 -> AMCLIB_Windmilling_SF/11
  f32AccPI/1 -> AMCLIB_Windmilling_SF/10
  u16NShiftI/1 -> AMCLIB_Windmilling_SF/9
  f32C1/1 -> AMCLIB_Windmilling_SF/8
  u16NShiftPI/1 -> AMCLIB_Windmilling_SF/7
  f32LowerLimit/1 -> AMCLIB_Windmilling_SF/6
  f32UpperLimit/1 -> AMCLIB_Windmilling_SF/5
  f32CC2sc/1 -> AMCLIB_Windmilling_SF/4
  f32CC1sc/1 -> AMCLIB_Windmilling_SF/3
  f32ADCMaxError/1 -> AMCLIB_Windmilling_SF/2
  pUabcIn/1 -> AMCLIB_Windmilling_SF/1

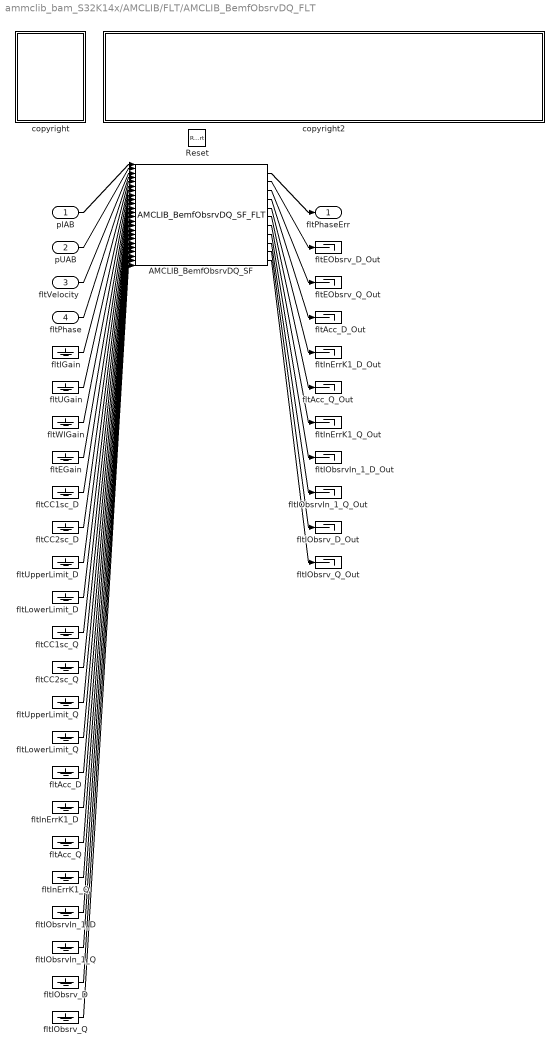
== system ammclib_bam_S32K14x/AMCLIB/FLT/AMCLIB_BemfObsrvDQ_FLT ==
  pIAB : Inport  OutDataTypeStr=Bus: SWLIBS_2Syst_FLT  BusOutputAsStruct=on
  pUAB : Inport  Port=2  OutDataTypeStr=Bus: SWLIBS_2Syst_FLT  BusOutputAsStruct=on
  fltVelocity : Inport  Port=3  OutDataTypeStr=single
  fltPhase : Inport  Port=4  OutDataTypeStr=single
  Reset : ResetPort  DisableCoverage=on
  AMCLIB_BemfObsrvDQ_SF : S-Function  FunctionName=AMCLIB_BemfObsrvDQ_SF_FLT  Parameters=showStates,resetStatesEnable,fltIGain,fltUGain,fltWIGain,fltEGain,fltCC1sc_D,fltCC2sc_D,fltUpperLimit_D,fltLowerLimit_D,fltCC1sc_Q,fltCC2sc_Q,fltUpperLimit_Q,fltLowerLimit_Q  SFunctionDeploymentMode=off  EnableBusSupport=off
  copyright : Subsystem
      mask Display: text(10,90,'FILE:');text(10,75,'DESRIPTION:');text(10,60,'COPYRIGHT:');text(10,45,'VERSION:');text(10,30,'DATE:')
  copyright2 : Subsystem
      mask Display: text(10,90,'AMCLIB_BemfObsrvDQ_BAM_FLT.mdl');text(10,75,'PMSM back-EMF observer DQ.');text(10,60,'NXP 2020');text(10,45,'1.0');text(10,30,'28-Mar-2020');
  fltAcc_D : Ground
  fltAcc_D_Out : Terminator
  fltAcc_Q : Ground
  fltAcc_Q_Out : Terminator
  fltCC1sc_D : Ground
  fltCC1sc_Q : Ground
  fltCC2sc_D : Ground
  fltCC2sc_Q : Ground
  fltEGain : Ground
  fltEObsrv_D_Out : Terminator
  fltEObsrv_Q_Out : Terminator
  fltIGain : Ground
  fltIObsrvIn_1_D : Ground
  fltIObsrvIn_1_D_Out : Terminator
  fltIObsrvIn_1_Q : Ground
  fltIObsrvIn_1_Q_Out : Terminator
  fltIObsrv_D : Ground
  fltIObsrv_D_Out : Terminator
  fltIObsrv_Q : Ground
  fltIObsrv_Q_Out : Terminator
  fltInErrK1_D : Ground
  fltInErrK1_D_Out : Terminator
  fltInErrK1_Q : Ground
  fltInErrK1_Q_Out : Terminator
  fltLowerLimit_D : Ground
  fltLowerLimit_Q : Ground
  fltUGain : Ground
  fltUpperLimit_D : Ground
  fltUpperLimit_Q : Ground
  fltWIGain : Ground
  fltPhaseErr : Outport
  wires:
  AMCLIB_BemfObsrvDQ_SF/11 -> fltIObsrv_Q_Out/1
  AMCLIB_BemfObsrvDQ_SF/10 -> fltIObsrv_D_Out/1
  AMCLIB_BemfObsrvDQ_SF/9 -> fltIObsrvIn_1_Q_Out/1
  AMCLIB_BemfObsrvDQ_SF/8 -> fltIObsrvIn_1_D_Out/1
  AMCLIB_BemfObsrvDQ_SF/7 -> fltInErrK1_Q_Out/1
  AMCLIB_BemfObsrvDQ_SF/6 -> fltAcc_Q_Out/1
  AMCLIB_BemfObsrvDQ_SF/5 -> fltInErrK1_D_Out/1
  AMCLIB_BemfObsrvDQ_SF/4 -> fltAcc_D_Out/1
  AMCLIB_BemfObsrvDQ_SF/3 -> fltEObsrv_Q_Out/1
  AMCLIB_BemfObsrvDQ_SF/2 -> fltEObsrv_D_Out/1
  AMCLIB_BemfObsrvDQ_SF/1 -> fltPhaseErr/1
  fltIObsrv_Q/1 -> AMCLIB_BemfObsrvDQ_SF/24
  fltIObsrv_D/1 -> AMCLIB_BemfObsrvDQ_SF/23
  fltIObsrvIn_1_Q/1 -> AMCLIB_BemfObsrvDQ_SF/22
  fltIObsrvIn_1_D/1 -> AMCLIB_BemfObsrvDQ_SF/21
  fltInErrK1_Q/1 -> AMCLIB_BemfObsrvDQ_SF/20
  fltAcc_Q/1 -> AMCLIB_BemfObsrvDQ_SF/19
  fltInErrK1_D/1 -> AMCLIB_BemfObsrvDQ_SF/18
  fltAcc_D/1 -> AMCLIB_BemfObsrvDQ_SF/17
  fltLowerLimit_Q/1 -> AMCLIB_BemfObsrvDQ_SF/16
  fltUpperLimit_Q/1 -> AMCLIB_BemfObsrvDQ_SF/15
  fltCC2sc_Q/1 -> AMCLIB_BemfObsrvDQ_SF/14
  fltCC1sc_Q/1 -> AMCLIB_BemfObsrvDQ_SF/13
  fltLowerLimit_D/1 -> AMCLIB_BemfObsrvDQ_SF/12
  fltUpperLimit_D/1 -> AMCLIB_BemfObsrvDQ_SF/11
  fltCC2sc_D/1 -> AMCLIB_BemfObsrvDQ_SF/10
  fltCC1sc_D/1 -> AMCLIB_BemfObsrvDQ_SF/9
  fltEGain/1 -> AMCLIB_BemfObsrvDQ_SF/8
  fltWIGain/1 -> AMCLIB_BemfObsrvDQ_SF/7
  fltUGain/1 -> AMCLIB_BemfObsrvDQ_SF/6
  fltIGain/1 -> AMCLIB_BemfObsrvDQ_SF/5
  fltPhase/1 -> AMCLIB_BemfObsrvDQ_SF/4
  fltVelocity/1 -> AMCLIB_BemfObsrvDQ_SF/3
  pUAB/1 -> AMCLIB_BemfObsrvDQ_SF/2
  pIAB/1 -> AMCLIB_BemfObsrvDQ_SF/1

== system ammclib_bam_S32K14x/AMCLIB/FLT/AMCLIB_CurrentLoop_FLT ==
  fltUDcBus : Inport  OutDataTypeStr=single
  pIDQReq : Inport  Port=2  OutDataTypeStr=Bus: SWLIBS_2Syst_FLT  BusOutputAsStruct=on
  pIDQFbck : Inport  Port=3  OutDataTypeStr=Bus: SWLIBS_2Syst_FLT  BusOutputAsStruct=on
  fltControllerPIrAWDOut_preset : Inport  Port=4  OutDataTypeStr=single
  fltControllerPIrAWQOut_preset : Inport  Port=5  OutDataTypeStr=single
  Reset : ResetPort  DisableCoverage=on
  AMCLIB_CurrentLoop_SF : S-Function  FunctionName=AMCLIB_CurrentLoop_SF_FLT  Parameters=showStates,resetStatesEnable,fltCC1sc_D,fltCC2sc_D,fltCC1sc_Q,fltCC2sc_Q  SFunctionDeploymentMode=off  EnableBusSupport=off
  copyright : Subsystem
      mask Display: text(10,90,'FILE:');text(10,75,'DESRIPTION:');text(10,60,'COPYRIGHT:');text(10,45,'VERSION:');text(10,30,'DATE:')
  copyright2 : Subsystem
      mask Display: text(10,90,'AMCLIB_CurrentLoop_BAM_FLT.mdl');text(10,75,'PMSM Current Loop.');text(10,60,'NXP 2020');text(10,45,'1.0');text(10,30,'28-Mar-2020');
  fltAcc_D : Ground
  fltAcc_D_Out : Terminator
  fltAcc_Q : Ground
  fltAcc_Q_Out : Terminator
  fltCC1sc_D : Ground
  fltCC1sc_Q : Ground
  fltCC2sc_D : Ground
  fltCC2sc_Q : Ground
  fltInErrK1_D : Ground
  fltInErrK1_D_Out : Terminator
  fltInErrK1_Q : Ground
  fltInErrK1_Q_Out : Terminator
  pUDQReq : Outport
  wires:
  AMCLIB_CurrentLoop_SF/5 -> fltInErrK1_Q_Out/1
  AMCLIB_CurrentLoop_SF/4 -> fltAcc_Q_Out/1
  AMCLIB_CurrentLoop_SF/3 -> fltInErrK1_D_Out/1
  AMCLIB_CurrentLoop_SF/2 -> fltAcc_D_Out/1
  AMCLIB_CurrentLoop_SF/1 -> pUDQReq/1
  fltInErrK1_Q/1 -> AMCLIB_CurrentLoop_SF/13
  fltAcc_Q/1 -> AMCLIB_CurrentLoop_SF/12
  fltInErrK1_D/1 -> AMCLIB_CurrentLoop_SF/11
  fltAcc_D/1 -> AMCLIB_CurrentLoop_SF/10
  fltCC2sc_Q/1 -> AMCLIB_CurrentLoop_SF/9
  fltCC1sc_Q/1 -> AMCLIB_CurrentLoop_SF/8
  fltCC2sc_D/1 -> AMCLIB_CurrentLoop_SF/7
  fltCC1sc_D/1 -> AMCLIB_CurrentLoop_SF/6
  fltControllerPIrAWQOut_preset/1 -> AMCLIB_CurrentLoop_SF/5
  fltControllerPIrAWDOut_preset/1 -> AMCLIB_CurrentLoop_SF/4
  pIDQFbck/1 -> AMCLIB_CurrentLoop_SF/3
  pIDQReq/1 -> AMCLIB_CurrentLoop_SF/2
  fltUDcBus/1 -> AMCLIB_CurrentLoop_SF/1

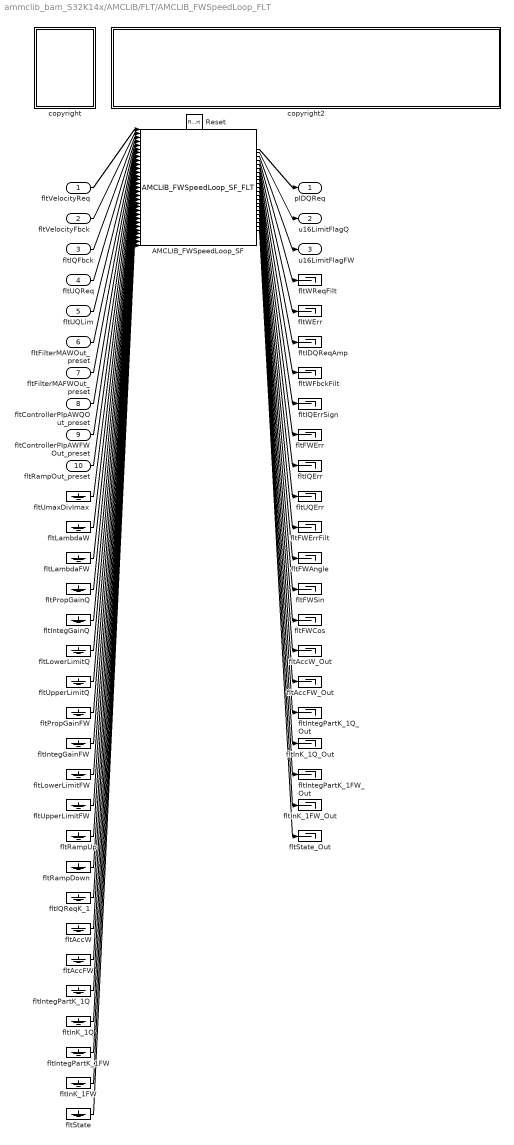
== system ammclib_bam_S32K14x/AMCLIB/FLT/AMCLIB_FWSpeedLoop_FLT ==
  fltVelocityReq : Inport  OutDataTypeStr=single
  fltVelocityFbck : Inport  Port=2  OutDataTypeStr=single
  fltIQFbck : Inport  Port=3  OutDataTypeStr=single
  fltUQReq : Inport  Port=4  OutDataTypeStr=single
  fltUQLim : Inport  Port=5  OutDataTypeStr=single
  fltFilterMAWOut_preset : Inport  Port=6  OutDataTypeStr=single
  fltFilterMAFWOut_preset : Inport  Port=7  OutDataTypeStr=single
  fltControllerPIpAWQOut_preset : Inport  Port=8  OutDataTypeStr=single
  fltControllerPIpAWFWOut_preset : Inport  Port=9  OutDataTypeStr=single
  fltRampOut_preset : Inport  Port=10  OutDataTypeStr=single
  Reset : ResetPort  DisableCoverage=on
  AMCLIB_FWSpeedLoop_SF : S-Function  FunctionName=AMCLIB_FWSpeedLoop_SF_FLT  Parameters=showStates,resetStatesEnable,showDebugOutputs,fltUmaxDivImax,fltLambdaW,fltLambdaFW,fltPropGainQ,fltIntegGainQ,fltLowerLimitQ,fltUpperLimitQ,fltPropGainFW,fltIntegGainFW,fltLowerLimitFW,fltUpperLimitFW,fltRampUp,fltRampDown  SFunctionDeploymentMode=off  EnableBusSupport=off
  copyright : Subsystem
      mask Display: text(10,90,'FILE:');text(10,75,'DESRIPTION:');text(10,60,'COPYRIGHT:');text(10,45,'VERSION:');text(10,30,'DATE:')
  copyright2 : Subsystem
      mask Display: text(10,90,'AMCLIB_FWSpeedLoop_BAM_FLT.mdl');text(10,75,'PMSM Speed Loop with Field Weakening.');text(10,60,'NXP 2020');text(10,45,'1.0');text(10,30,'28-Mar-2020');
  fltAccFW : Ground
  fltAccFW_Out : Terminator
  fltAccW : Ground
  fltAccW_Out : Terminator
  fltFWAngle : Terminator
  fltFWCos : Terminator
  fltFWErr : Terminator
  fltFWErrFilt : Terminator
  fltFWSin : Terminator
  fltIDQReqAmp : Terminator
  fltIQErr : Terminator
  fltIQErrSign : Terminator
  fltIQReqK_1 : Ground
  fltInK_1FW : Ground
  fltInK_1FW_Out : Terminator
  fltInK_1Q : Ground
  fltInK_1Q_Out : Terminator
  fltIntegGainFW : Ground
  fltIntegGainQ : Ground
  fltIntegPartK_1FW : Ground
  fltIntegPartK_1FW_Out : Terminator
  fltIntegPartK_1Q : Ground
  fltIntegPartK_1Q_Out : Terminator
  fltLambdaFW : Ground
  fltLambdaW : Ground
  fltLowerLimitFW : Ground
  fltLowerLimitQ : Ground
  fltPropGainFW : Ground
  fltPropGainQ : Ground
  fltRampDown : Ground
  fltRampUp : Ground
  fltState : Ground
  fltState_Out : Terminator
  fltUQErr : Terminator
  fltUmaxDivImax : Ground
  fltUpperLimitFW : Ground
  fltUpperLimitQ : Ground
  fltWErr : Terminator
  fltWFbckFilt : Terminator
  fltWReqFilt : Terminator
  pIDQReq : Outport
  u16LimitFlagQ : Outport  Port=2
  u16LimitFlagFW : Outport  Port=3
  wires:
  AMCLIB_FWSpeedLoop_SF/22 -> fltState_Out/1
  AMCLIB_FWSpeedLoop_SF/21 -> fltInK_1FW_Out/1
  AMCLIB_FWSpeedLoop_SF/20 -> fltIntegPartK_1FW_Out/1
  AMCLIB_FWSpeedLoop_SF/19 -> fltInK_1Q_Out/1
  AMCLIB_FWSpeedLoop_SF/18 -> fltIntegPartK_1Q_Out/1
  AMCLIB_FWSpeedLoop_SF/17 -> fltAccFW_Out/1
  AMCLIB_FWSpeedLoop_SF/16 -> fltAccW_Out/1
  AMCLIB_FWSpeedLoop_SF/15 -> fltFWCos/1
  AMCLIB_FWSpeedLoop_SF/14 -> fltFWSin/1
  AMCLIB_FWSpeedLoop_SF/13 -> fltFWAngle/1
  AMCLIB_FWSpeedLoop_SF/12 -> fltFWErrFilt/1
  AMCLIB_FWSpeedLoop_SF/11 -> fltUQErr/1
  AMCLIB_FWSpeedLoop_SF/10 -> fltIQErr/1
  AMCLIB_FWSpeedLoop_SF/9 -> fltFWErr/1
  AMCLIB_FWSpeedLoop_SF/8 -> fltIQErrSign/1
  AMCLIB_FWSpeedLoop_SF/7 -> fltWFbckFilt/1
  AMCLIB_FWSpeedLoop_SF/6 -> fltIDQReqAmp/1
  AMCLIB_FWSpeedLoop_SF/5 -> fltWErr/1
  AMCLIB_FWSpeedLoop_SF/4 -> fltWReqFilt/1
  AMCLIB_FWSpeedLoop_SF/3 -> u16LimitFlagFW/1
  AMCLIB_FWSpeedLoop_SF/2 -> u16LimitFlagQ/1
  AMCLIB_FWSpeedLoop_SF/1 -> pIDQReq/1
  fltState/1 -> AMCLIB_FWSpeedLoop_SF/31
  fltInK_1FW/1 -> AMCLIB_FWSpeedLoop_SF/30
  fltIntegPartK_1FW/1 -> AMCLIB_FWSpeedLoop_SF/29
  fltInK_1Q/1 -> AMCLIB_FWSpeedLoop_SF/28
  fltIntegPartK_1Q/1 -> AMCLIB_FWSpeedLoop_SF/27
  fltAccFW/1 -> AMCLIB_FWSpeedLoop_SF/26
  fltAccW/1 -> AMCLIB_FWSpeedLoop_SF/25
  fltIQReqK_1/1 -> AMCLIB_FWSpeedLoop_SF/24
  fltRampDown/1 -> AMCLIB_FWSpeedLoop_SF/23
  fltRampUp/1 -> AMCLIB_FWSpeedLoop_SF/22
  fltUpperLimitFW/1 -> AMCLIB_FWSpeedLoop_SF/21
  fltLowerLimitFW/1 -> AMCLIB_FWSpeedLoop_SF/20
  fltIntegGainFW/1 -> AMCLIB_FWSpeedLoop_SF/19
  fltPropGainFW/1 -> AMCLIB_FWSpeedLoop_SF/18
  fltUpperLimitQ/1 -> AMCLIB_FWSpeedLoop_SF/17
  fltLowerLimitQ/1 -> AMCLIB_FWSpeedLoop_SF/16
  fltIntegGainQ/1 -> AMCLIB_FWSpeedLoop_SF/15
  fltPropGainQ/1 -> AMCLIB_FWSpeedLoop_SF/14
  fltLambdaFW/1 -> AMCLIB_FWSpeedLoop_SF/13
  fltLambdaW/1 -> AMCLIB_FWSpeedLoop_SF/12
  fltUmaxDivImax/1 -> AMCLIB_FWSpeedLoop_SF/11
  fltRampOut_preset/1 -> AMCLIB_FWSpeedLoop_SF/10
  fltControllerPIpAWFWOut_preset/1 -> AMCLIB_FWSpeedLoop_SF/9
  fltControllerPIpAWQOut_preset/1 -> AMCLIB_FWSpeedLoop_SF/8
  fltFilterMAFWOut_preset/1 -> AMCLIB_FWSpeedLoop_SF/7
  fltFilterMAWOut_preset/1 -> AMCLIB_FWSpeedLoop_SF/6
  fltUQLim/1 -> AMCLIB_FWSpeedLoop_SF/5
  fltUQReq/1 -> AMCLIB_FWSpeedLoop_SF/4
  fltIQFbck/1 -> AMCLIB_FWSpeedLoop_SF/3
  fltVelocityFbck/1 -> AMCLIB_FWSpeedLoop_SF/2
  fltVelocityReq/1 -> AMCLIB_FWSpeedLoop_SF/1

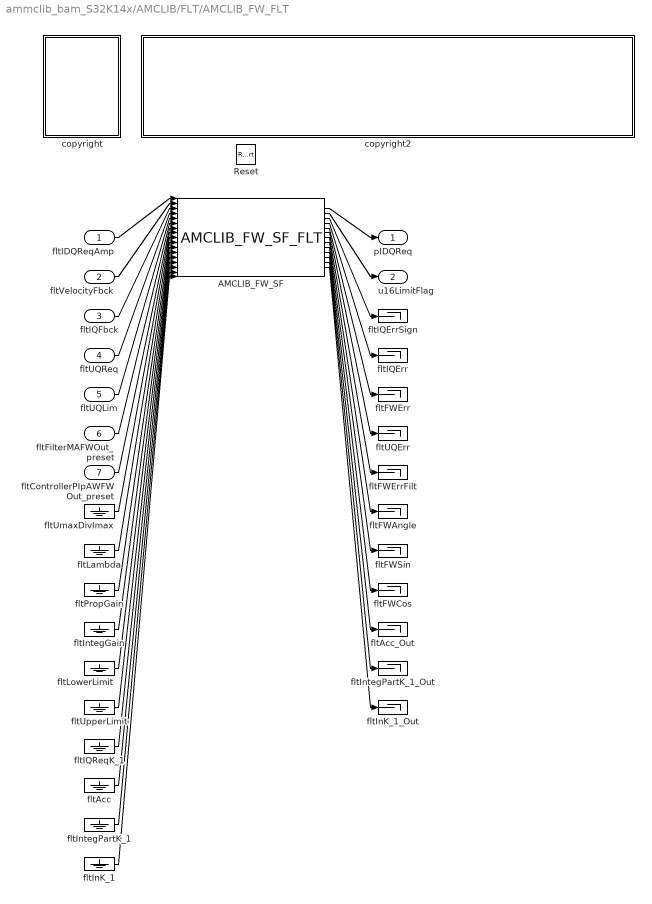
== system ammclib_bam_S32K14x/AMCLIB/FLT/AMCLIB_FW_FLT ==
  fltIDQReqAmp : Inport  OutDataTypeStr=single
  fltVelocityFbck : Inport  Port=2  OutDataTypeStr=single
  fltIQFbck : Inport  Port=3  OutDataTypeStr=single
  fltUQReq : Inport  Port=4  OutDataTypeStr=single
  fltUQLim : Inport  Port=5  OutDataTypeStr=single
  fltFilterMAFWOut_preset : Inport  Port=6  OutDataTypeStr=single
  fltControllerPIpAWFWOut_preset : Inport  Port=7  OutDataTypeStr=single
  Reset : ResetPort  DisableCoverage=on
  AMCLIB_FW_SF : S-Function  FunctionName=AMCLIB_FW_SF_FLT  Parameters=showStates,resetStatesEnable,showDebugOutputs,fltUmaxDivImax,fltLambda,fltPropGain,fltIntegGain,fltLowerLimit,fltUpperLimit  SFunctionDeploymentMode=off  EnableBusSupport=off
  copyright : Subsystem
      mask Display: text(10,90,'FILE:');text(10,75,'DESRIPTION:');text(10,60,'COPYRIGHT:');text(10,45,'VERSION:');text(10,30,'DATE:')
  copyright2 : Subsystem
      mask Display: text(10,90,'AMCLIB_FW_BAM_FLT.mdl');text(10,75,'PMSM Field Weakening Controller');text(10,60,'NXP 2020');text(10,45,'1.0');text(10,30,'28-Mar-2020');
  fltAcc : Ground
  fltAcc_Out : Terminator
  fltFWAngle : Terminator
  fltFWCos : Terminator
  fltFWErr : Terminator
  fltFWErrFilt : Terminator
  fltFWSin : Terminator
  fltIQErr : Terminator
  fltIQErrSign : Terminator
  fltIQReqK_1 : Ground
  fltInK_1 : Ground
  fltInK_1_Out : Terminator
  fltIntegGain : Ground
  fltIntegPartK_1 : Ground
  fltIntegPartK_1_Out : Terminator
  fltLambda : Ground
  fltLowerLimit : Ground
  fltPropGain : Ground
  fltUQErr : Terminator
  fltUmaxDivImax : Ground
  fltUpperLimit : Ground
  pIDQReq : Outport
  u16LimitFlag : Outport  Port=2
  wires:
  AMCLIB_FW_SF/13 -> fltInK_1_Out/1
  AMCLIB_FW_SF/12 -> fltIntegPartK_1_Out/1
  AMCLIB_FW_SF/11 -> fltAcc_Out/1
  AMCLIB_FW_SF/10 -> fltFWCos/1
  AMCLIB_FW_SF/9 -> fltFWSin/1
  AMCLIB_FW_SF/8 -> fltFWAngle/1
  AMCLIB_FW_SF/7 -> fltFWErrFilt/1
  AMCLIB_FW_SF/6 -> fltUQErr/1
  AMCLIB_FW_SF/5 -> fltFWErr/1
  AMCLIB_FW_SF/4 -> fltIQErr/1
  AMCLIB_FW_SF/3 -> fltIQErrSign/1
  AMCLIB_FW_SF/2 -> u16LimitFlag/1
  AMCLIB_FW_SF/1 -> pIDQReq/1
  fltInK_1/1 -> AMCLIB_FW_SF/17
  fltIntegPartK_1/1 -> AMCLIB_FW_SF/16
  fltAcc/1 -> AMCLIB_FW_SF/15
  fltIQReqK_1/1 -> AMCLIB_FW_SF/14
  fltUpperLimit/1 -> AMCLIB_FW_SF/13
  fltLowerLimit/1 -> AMCLIB_FW_SF/12
  fltIntegGain/1 -> AMCLIB_FW_SF/11
  fltPropGain/1 -> AMCLIB_FW_SF/10
  fltLambda/1 -> AMCLIB_FW_SF/9
  fltUmaxDivImax/1 -> AMCLIB_FW_SF/8
  fltControllerPIpAWFWOut_preset/1 -> AMCLIB_FW_SF/7
  fltFilterMAFWOut_preset/1 -> AMCLIB_FW_SF/6
  fltUQLim/1 -> AMCLIB_FW_SF/5
  fltUQReq/1 -> AMCLIB_FW_SF/4
  fltIQFbck/1 -> AMCLIB_FW_SF/3
  fltVelocityFbck/1 -> AMCLIB_FW_SF/2
  fltIDQReqAmp/1 -> AMCLIB_FW_SF/1

== system ammclib_bam_S32K14x/AMCLIB/FLT/AMCLIB_SpeedLoop_FLT ==
  fltVelocityReq : Inport  OutDataTypeStr=single
  fltVelocityFbck : Inport  Port=2  OutDataTypeStr=single
  fltFilterMAWOut_preset : Inport  Port=3  OutDataTypeStr=single
  fltControllerPIpAWQOut_preset : Inport  Port=4  OutDataTypeStr=single
  fltRampOut_preset : Inport  Port=5  OutDataTypeStr=single
  Reset : ResetPort  DisableCoverage=on
  AMCLIB_SpeedLoop_SF : S-Function  FunctionName=AMCLIB_SpeedLoop_SF_FLT  Parameters=showStates,resetStatesEnable,showDebugOutputs,fltLambdaW,fltPropGainQ,fltIntegGainQ,fltLowerLimitQ,fltUpperLimitQ,fltRampUp,fltRampDown  SFunctionDeploymentMode=off  EnableBusSupport=off
  copyright : Subsystem
      mask Display: text(10,90,'FILE:');text(10,75,'DESRIPTION:');text(10,60,'COPYRIGHT:');text(10,45,'VERSION:');text(10,30,'DATE:')
  copyright2 : Subsystem
      mask Display: text(10,90,'AMCLIB_SpeedLoop_BAM_FLT.mdl');text(10,75,'PMSM Speed Loop Controller.');text(10,60,'NXP 2020');text(10,45,'1.0');text(10,30,'28-Mar-2020');
  fltAccW : Ground
  fltAccW_Out : Terminator
  fltInK_1Q : Ground
  fltInK_1Q_Out : Terminator
  fltIntegGainQ : Ground
  fltIntegPartK_1Q : Ground
  fltIntegPartK_1Q_Out : Terminator
  fltLambdaW : Ground
  fltLowerLimitQ : Ground
  fltPropGainQ : Ground
  fltRampDown : Ground
  fltRampUp : Ground
  fltState : Ground
  fltState_Out : Terminator
  fltUpperLimitQ : Ground
  fltWErr : Terminator
  fltWFbckFilt : Terminator
  fltWReqFilt : Terminator
  pIDQReq : Outport
  u16LimitFlagQ : Outport  Port=2
  wires:
  AMCLIB_SpeedLoop_SF/9 -> fltState_Out/1
  AMCLIB_SpeedLoop_SF/8 -> fltInK_1Q_Out/1
  AMCLIB_SpeedLoop_SF/7 -> fltIntegPartK_1Q_Out/1
  AMCLIB_SpeedLoop_SF/6 -> fltAccW_Out/1
  AMCLIB_SpeedLoop_SF/5 -> fltWFbckFilt/1
  AMCLIB_SpeedLoop_SF/4 -> fltWErr/1
  AMCLIB_SpeedLoop_SF/3 -> fltWReqFilt/1
  AMCLIB_SpeedLoop_SF/2 -> u16LimitFlagQ/1
  AMCLIB_SpeedLoop_SF/1 -> pIDQReq/1
  fltState/1 -> AMCLIB_SpeedLoop_SF/16
  fltInK_1Q/1 -> AMCLIB_SpeedLoop_SF/15
  fltIntegPartK_1Q/1 -> AMCLIB_SpeedLoop_SF/14
  fltAccW/1 -> AMCLIB_SpeedLoop_SF/13
  fltRampDown/1 -> AMCLIB_SpeedLoop_SF/12
  fltRampUp/1 -> AMCLIB_SpeedLoop_SF/11
  fltUpperLimitQ/1 -> AMCLIB_SpeedLoop_SF/10
  fltLowerLimitQ/1 -> AMCLIB_SpeedLoop_SF/9
  fltIntegGainQ/1 -> AMCLIB_SpeedLoop_SF/8
  fltPropGainQ/1 -> AMCLIB_SpeedLoop_SF/7
  fltLambdaW/1 -> AMCLIB_SpeedLoop_SF/6
  fltRampOut_preset/1 -> AMCLIB_SpeedLoop_SF/5
  fltControllerPIpAWQOut_preset/1 -> AMCLIB_SpeedLoop_SF/4
  fltFilterMAWOut_preset/1 -> AMCLIB_SpeedLoop_SF/3
  fltVelocityFbck/1 -> AMCLIB_SpeedLoop_SF/2
  fltVelocityReq/1 -> AMCLIB_SpeedLoop_SF/1

== system ammclib_bam_S32K14x/AMCLIB/FLT/AMCLIB_TrackObsrv_FLT ==
  fltPhaseErr : Inport  OutDataTypeStr=single
  fltVelocityOut_preset : Inport  Port=2  OutDataTypeStr=single
  fltPosOut_preset : Inport  Port=3  OutDataTypeStr=single
  Reset : ResetPort  DisableCoverage=on
  AMCLIB_TrackObsrv_SF : S-Function  FunctionName=AMCLIB_TrackObsrv_SF_FLT  Parameters=showStates,resetStatesEnable,fltCC1sc,fltCC2sc,fltUpperLimit,fltLowerLimit,fltC1  SFunctionDeploymentMode=off  EnableBusSupport=off
  copyright : Subsystem
      mask Display: text(10,90,'FILE:');text(10,75,'DESRIPTION:');text(10,60,'COPYRIGHT:');text(10,45,'VERSION:');text(10,30,'DATE:')
  copyright2 : Subsystem
      mask Display: text(10,90,'AMCLIB_TrackObsrv_BAM_FLT.mdl');text(10,75,'Tracking observer');text(10,60,'NXP 2020');text(10,45,'1.0');text(10,30,'28-Mar-2020');
  fltAcc : Ground
  fltAcc_Out : Terminator
  fltC1 : Ground
  fltCC1 : Ground
  fltCC2 : Ground
  fltInErrK1 : Ground
  fltInErrK1_Out : Terminator
  fltInK1 : Ground
  fltInK1_Out : Terminator
  fltLowerLimit : Ground
  fltState : Ground
  fltState_Out : Terminator
  fltUpperLimit : Ground
  pPosEst : Outport
  pVelocityEst : Outport  Port=2
  wires:
  AMCLIB_TrackObsrv_SF/6 -> fltInK1_Out/1
  AMCLIB_TrackObsrv_SF/5 -> fltState_Out/1
  AMCLIB_TrackObsrv_SF/4 -> fltInErrK1_Out/1
  AMCLIB_TrackObsrv_SF/3 -> fltAcc_Out/1
  AMCLIB_TrackObsrv_SF/2 -> pVelocityEst/1
  AMCLIB_TrackObsrv_SF/1 -> pPosEst/1
  fltInK1/1 -> AMCLIB_TrackObsrv_SF/12
  fltState/1 -> AMCLIB_TrackObsrv_SF/11
  fltInErrK1/1 -> AMCLIB_TrackObsrv_SF/10
  fltAcc/1 -> AMCLIB_TrackObsrv_SF/9
  fltC1/1 -> AMCLIB_TrackObsrv_SF/8
  fltLowerLimit/1 -> AMCLIB_TrackObsrv_SF/7
  fltUpperLimit/1 -> AMCLIB_TrackObsrv_SF/6
  fltCC2/1 -> AMCLIB_TrackObsrv_SF/5
  fltCC1/1 -> AMCLIB_TrackObsrv_SF/4
  fltPosOut_preset/1 -> AMCLIB_TrackObsrv_SF/3
  fltVelocityOut_preset/1 -> AMCLIB_TrackObsrv_SF/2
  fltPhaseErr/1 -> AMCLIB_TrackObsrv_SF/1
